simulink model "TenBots"  (R2016b)
settings: Solver=ode45  StartTime=0.0  StopTime=40  RelTol=1e-3  EnableMultiTasking=on
libraries: simulink x3
settings Model: Creator=Chris  LastModifiedBy=Syd
settings DataIOCC: LimitDataPoints=on  SaveFormat=Array
settings OptimizationCC: LifeSpan=inf
settings DebuggingCC: UnderspecifiedInitializationDetection=Classic  MergeDetectMultiDrivingBlocksExec=none  SolverPrmCheckMsg=warning  SFUnexpectedBacktrackingDiag=warning  SFNoUnconditionalDefaultTransitionDiag=warning  SFExecutionAtInitializationDiag=none
settings HardwareCC: ProdBitPerPointer=32  ProdBitPerSizeT=32  ProdBitPerPtrDiffT=32  ProdLargestAtomicFloat=None  ProdIntDivRoundTo=Undefined  ProdEndianess=Unspecified  ProdWordSize=32  ProdHWDeviceType=32-bit Generic
settings ModelReferenceCC: PropagateSignalLabelsOutOfModel=off
settings GRTTargetCC: TargetLangStandard=C89/C90 (ANSI)  GeneratePreprocessorConditionals=Disable all
settings ConfigComp: CovMetricSettings=dw  CovHtmlReporting=on  CovSaveCumulativeToWorkspaceVar=on  CovSaveSingleToWorkspaceVar=on  CovExternalEMLEnable=off

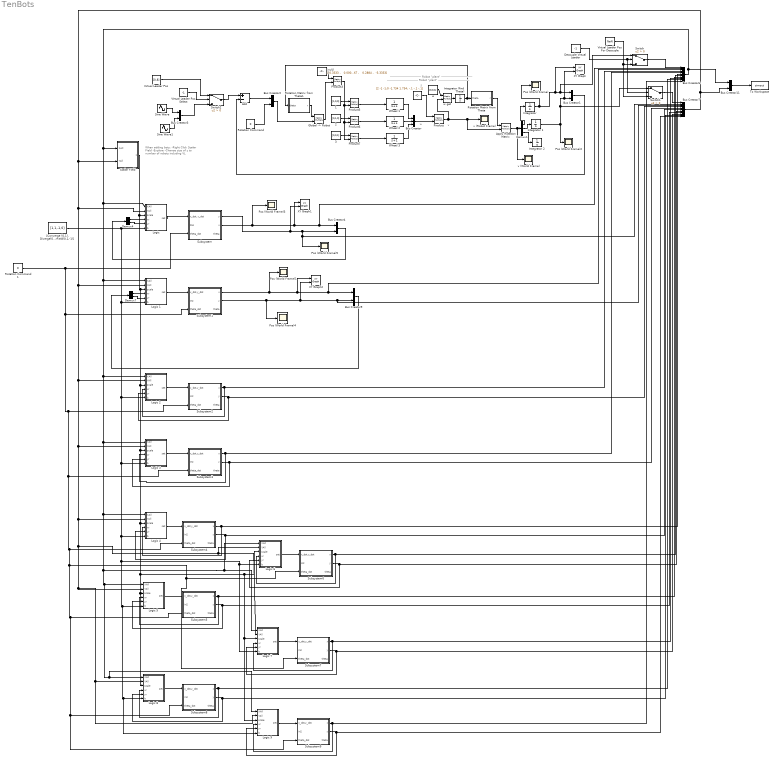
== system TenBots ==
  note: When adding bots:
      | -Right Click Scalar Field
      | -Explore
      | -Change size of z to number of robots including VL
  note: ------------------------------- Robot "plant" -------------------------------
  note: v
  note: w
  note: ------------------------------- Robot "plant" -------------------------------
  1 : Constant  Value=[1,0,0]  VectorParams1D=off
  2 : Constant  Value=[0,1,0]  VectorParams1D=off
  3 : Constant  Value=[0,0,1]  VectorParams1D=off
  Add : Sum  Inputs=+-
  Apply Rotation Matrix : Product  Multiplication=Matrix(*)
  Bus Creator : BusCreator  Inputs=3
  Bus Creator{1..4,9,11} (6 alike) : BusCreator  Inputs=2
  Bus Creator6 : BusCreator  Inputs=11
  Bus Creator7 : BusCreator  Inputs=11
  Decouple Virtual Leader : Constant  Value=-1
  Demux1 : Demux  Outputs=3
  Demux4 : Demux  Outputs=2
  Demux7 : Demux  Outputs=2
  "Global -> Robot" : Product  Multiplication=Matrix(*)
  "Integrator " : Integrator
  Integrator (find Theta) : Integrator
  Integrator 1 : Integrator
  Integrator 2 : Integrator  InitialCondition=1
  J : Constant  Value=[2 -1 -1;0 -1.734 1.734; -.1 -.1 -.1]
  "Logic " : MATLAB Function  TreatAsAtomicUnit=on
  Logic 1 : MATLAB Function  TreatAsAtomicUnit=on
  Logic 2 : MATLAB Function  TreatAsAtomicUnit=on
  Logic 3 : MATLAB Function  TreatAsAtomicUnit=on
  Logic 4 : MATLAB Function  TreatAsAtomicUnit=on
  Logic 5 : MATLAB Function  TreatAsAtomicUnit=on
  Logic 6 : MATLAB Function  TreatAsAtomicUnit=on
  Logic 7 : MATLAB Function  TreatAsAtomicUnit=on
  Logic 8 : MATLAB Function  TreatAsAtomicUnit=on
  Logic 9 : MATLAB Function  TreatAsAtomicUnit=on
  Pos (World Frame){,1..5} (6 alike) : Scope
  Product{,3,5..7} (5 alike) : Product  Multiplication=Matrix(*)
  Rotation Command : Constant  Value=0
  Rotation Command 1 : Constant  Value=0
  Rotation Matrix from Theta : MATLAB Function  TreatAsAtomicUnit=on
  Rotation Matrix from Theta1 : MATLAB Function  TreatAsAtomicUnit=on
  Scalar Field : MATLAB Function  TreatAsAtomicUnit=on
  Sine Wave : Sin  Amplitude=4  SampleTime=0
  Sine Wave1 : Sin  Phase=pi/2  SampleTime=0
  Subsystem : Subsystem
  Subsystem1 : Subsystem
  Subsystem2 : Subsystem
  Subsystem3 : Subsystem
  Subsystem4 : Subsystem
  Subsystem5 : Subsystem
  Subsystem6 : Subsystem
  Subsystem7 : Subsystem
  Subsystem8 : Subsystem
  Subsystem9 : Subsystem
  Switch : Switch  Criteria=u2 > Threshold
  Switch1 : Switch  Criteria=u2 > Threshold
  Switch2 : Switch  Criteria=u2 > Threshold
  To Workspace : ToWorkspace  VariableName=simout  SampleTime=-1
  VIrtual Leader Pos Select : Constant  Value=-1
  Virtual Leader Pos : Constant  Value=[0,8]
  Virtual Leader Pos For Decouple : Constant  Value=NaN
  Wheel 1 : TransferFcn  Denominator=[1 1]
  Wheel 2 : TransferFcn  Denominator=[1 1]
  Wheel 3 : TransferFcn  Denominator=[1 1]  ContinuousStateAttributes='orientation'
  XY Graph : simulink/Sinks/XY Graph  xmin=-1  xmax=3  ymin=-1  ymax=11  st=.1
  XY Graph1 : simulink/Sinks/XY Graph  xmin=-1  xmax=3  ymin=-1  ymax=10  st=.1
  XY Graph2 : simulink/Sinks/XY Graph  xmin=-1  xmax=3  ymin=-1  ymax=10  st=.1
  "[Converge (0,1), Diverge(0,1), Orbit(0,1,-1), ScalarField(0,1,-1)]" : Constant  Value=[1,1,-1,0]
  inv(J) : Constant  Value=|
      | [ 0.3333 ,   0.0000 ,  -3.3333
      |  ;  -0.1667  , -0.2884  , -3.3333
      |  ;  -0.1667 ,   0.2884 ,  -3.3333]
  v (Robot Frame) : Scope
  v (World Frame) : Scope
  w : Constant  Value=[0,0,1]  VectorParams1D=off
  w get : Product  Multiplication=Matrix(*)
  wires:
  Wheel 1/1 -> Bus Creator/1
  Wheel 3/1 -> Bus Creator/3
  J/1 -> Product/1
  Product/1 -> Apply Rotation Matrix/2, v (Robot Frame)/1, w get/2
  Product5/1 -> Wheel 1/1
  Product6/1 -> Wheel 2/1
  Product7/1 -> Wheel 3/1
  w get/1 -> Integrator (find Theta)/1
  Rotation Matrix from Theta/1(r) -> Apply Rotation Matrix/1
  Apply Rotation Matrix/1 -> Demux1/1, v (World Frame)/1
  inv(J)/1 -> Product3/1
  w/1 -> w get/1
  1/1 -> Product5/1
  Product3/1 -> Product6/2, Product7/2, Product5/2
  3/1 -> Product7/1
  2/1 -> Product6/1
  "Global -> Robot"/1 -> Product3/2
  Integrator (find Theta)/1 -> Rotation Matrix from Theta1/1(theta), Rotation Matrix from Theta/1(theta)
  Rotation Matrix from Theta1/1(r) -> "Global -> Robot"/1
  Bus Creator2/1 -> "Global -> Robot"/2
  Bus Creator/1 -> Product/2
  Wheel 2/1 -> Bus Creator/2
  Virtual Leader Pos/1 -> Switch2/1
  Integrator 1/1 -> Switch1/1, XY Graph/2, Bus Creator1/2, Pos (World Frame)2/1
  "Integrator "/1 -> XY Graph/1, Switch/1, Bus Creator1/1, Pos (World Frame)/1
  Bus Creator1/1 -> Add/2
  Add/1 -> Bus Creator2/1
  Demux1/1 -> "Integrator "/1
  Demux1/2 -> Integrator 1/1
  Demux1/3 -> Integrator 2/1
  Rotation Command/1 -> Bus Creator2/2
  Bus Creator4/1 -> Demux4/1
  Demux4/1 -> "Logic "/4(xr)
  Demux4/2 -> "Logic "/5(yr)
  Bus Creator9/1 -> Demux7/1
  Demux7/1 -> Logic 1/4(xr)
  Demux7/2 -> Logic 1/5(yr)
  Bus Creator11/1 -> To Workspace/1
  Subsystem/1(y) -> Bus Creator7/2, Pos (World Frame)5/1, Bus Creator4/2, XY Graph1/2
  Subsystem/2(x) -> Pos (World Frame)3/1, Bus Creator4/1, Bus Creator6/2, XY Graph1/1
  "Logic "/1(set) -> Subsystem/1("x_dot, y_dot")
  Subsystem1/1(x) -> Bus Creator9/1, Bus Creator6/3, XY Graph2/1, Pos (World Frame)1/1
  Subsystem1/2(y) -> Pos (World Frame)4/1, Bus Creator7/3, Bus Creator9/2, XY Graph2/2
  Logic 1/1(set) -> Subsystem1/1(x_dot,y_dot)
  Logic 2/1(set) -> Subsystem2/1(x_dot,y_dot)
  Subsystem2/1(x) -> Bus Creator6/4, Logic 2/4(xr)
  Subsystem2/2(y) -> Bus Creator7/4, Logic 2/5(yr)
  Logic 3/1(set) -> Subsystem3/1(x_dot,y_dot)
  Subsystem3/1(x) -> Logic 3/4(xr), Bus Creator6/5
  Subsystem3/2(y) -> Bus Creator7/5, Logic 3/5(yr)
  Switch/1 -> Bus Creator6/1
  Switch1/1 -> Bus Creator7/1
  Decouple Virtual Leader/1 -> Switch1/2, Switch/2
  Virtual Leader Pos For Decouple/1 -> Switch1/3, Switch/3
  Logic 4/1(set) -> Subsystem4/1(x_dot,y_dot)
  Subsystem4/1(x) -> Bus Creator6/6, Logic 4/4(xr)
  Subsystem4/2(y) -> Bus Creator7/6, Logic 4/5(yr)
  Logic 5/1(set) -> Subsystem5/1(x_dot,y_dot)
  Subsystem5/1(x) -> Bus Creator6/8, Logic 5/4(xr)
  Subsystem5/2(y) -> Bus Creator7/8, Logic 5/5(yr)
  Logic 6/1(set) -> Subsystem6/1(x_dot,y_dot)
  Subsystem6/1(x) -> Bus Creator6/7, Logic 6/4(xr)
  Subsystem6/2(y) -> Bus Creator7/7, Logic 6/5(yr)
  Logic 7/1(set) -> Subsystem7/1(x_dot,y_dot)
  Subsystem7/1(x) -> Bus Creator6/9, Logic 7/4(xr)
  Subsystem7/2(y) -> Bus Creator7/9, Logic 7/5(yr)
  Logic 8/1(set) -> Subsystem8/1(x_dot,y_dot)
  Subsystem8/1(x) -> Bus Creator6/10, Logic 8/4(xr)
  Subsystem8/2(y) -> Bus Creator7/10, Logic 8/5(yr)
  Bus Creator6/1 -> Bus Creator11/1, "Logic "/1(XAll), Logic 7/1(XAll), Logic 6/1(XAll), Logic 9/1(XAll), Logic 8/1(XAll), Logic 5/1(XAll), Logic 4/1(XAll), Logic 3/1(XAll), Logic 2/1(XAll), Logic 1/1(XAll), Scalar Field/1(XAll)
  Bus Creator7/1 -> Bus Creator11/2, "Logic "/2(YAll), Logic 7/2(YAll), Logic 6/2(YAll), Logic 9/2(YAll), Logic 8/2(YAll), Logic 5/2(YAll), Logic 4/2(YAll), Logic 3/2(YAll), Logic 2/2(YAll), Logic 1/2(YAll), Scalar Field/2(YAll)
  "[Converge (0,1), Diverge(0,1), Orbit(0,1,-1), ScalarField(0,1,-1)]"/1 -> "Logic "/6(b), Logic 2/6(b), Logic 7/6(b), Logic 6/6(b), Logic 9/6(b), Logic 8/6(b), Logic 5/6(b), Logic 4/6(b), Logic 3/6(b), Logic 1/6(b)
  Scalar Field/1(z) -> "Logic "/3(scale), Logic 9/3(scale), Logic 7/3(scale), Logic 6/3(scale), Logic 8/3(scale), Logic 5/3(scale), Logic 4/3(scale), Logic 3/3(scale), Logic 2/3(scale), Logic 1/3(scale)
  Logic 9/1(set) -> Subsystem9/1(x_dot,y_dot)
  Rotation Command 1/1 -> Subsystem7/3(theta_dot), Subsystem6/3(theta_dot), Subsystem9/3(theta_dot), Subsystem8/3(theta_dot), Subsystem5/3(theta_dot), Subsystem4/3(theta_dot), Subsystem3/3(theta_dot), Subsystem2/3(theta_dot), Subsystem1/3(theta_dot), Subsystem/3(theta_dot)
  Subsystem9/1(x) -> Bus Creator6/11, Logic 9/4(xr)
  Subsystem9/2(y) -> Bus Creator7/11, Logic 9/5(yr)
  Sine Wave/1 -> Bus Creator3/1
  Sine Wave1/1 -> Bus Creator3/2
  Switch2/1 -> Add/1
  Bus Creator3/1 -> Switch2/3
  VIrtual Leader Pos Select/1 -> Switch2/2

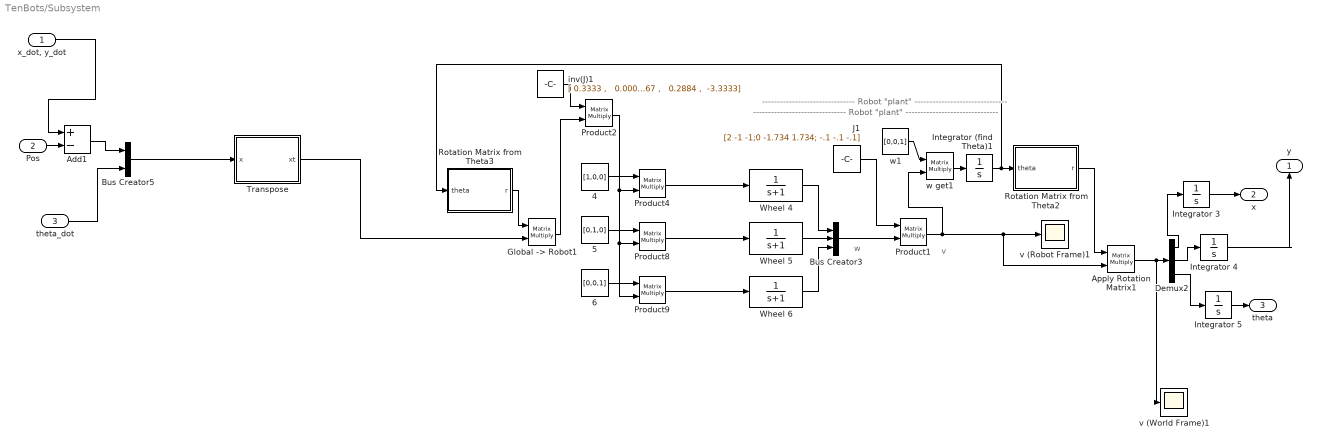
== system TenBots/Subsystem ==
  note: ------------------------------- Robot "plant" -------------------------------
  note: v
  note: w
  note: ------------------------------- Robot "plant" -------------------------------
  "x_dot, y_dot" : Inport
  Pos : Inport  Port=2
  theta_dot : Inport  Port=3
  4 : Constant  Value=[1,0,0]  VectorParams1D=off
  5 : Constant  Value=[0,1,0]  VectorParams1D=off
  6 : Constant  Value=[0,0,1]  VectorParams1D=off
  Add1 : Sum  Inputs=+-
  Apply Rotation Matrix1 : Product  Multiplication=Matrix(*)
  Bus Creator3 : BusCreator  Inputs=3
  Bus Creator5 : BusCreator  Inputs=2
  Demux2 : Demux  Outputs=3
  "Global -> Robot1" : Product  Multiplication=Matrix(*)
  Integrator (find Theta)1 : Integrator
  Integrator 3 : Integrator  InitialCondition=1
  Integrator 4 : Integrator  InitialCondition=1
  Integrator 5 : Integrator  InitialCondition=1
  J1 : Constant  Value=[2 -1 -1;0 -1.734 1.734; -.1 -.1 -.1]
  Product{1..2,4,8..9} (5 alike) : Product  Multiplication=Matrix(*)
  Rotation Matrix from Theta2 : MATLAB Function  TreatAsAtomicUnit=on
  Rotation Matrix from Theta3 : MATLAB Function  TreatAsAtomicUnit=on
  Transpose : MATLAB Function  TreatAsAtomicUnit=on
  Wheel 4 : TransferFcn  Denominator=[1 1]
  Wheel 5 : TransferFcn  Denominator=[1 1]
  Wheel 6 : TransferFcn  Denominator=[1 1]  ContinuousStateAttributes='orientation'
  inv(J)1 : Constant  Value=|
      | [ 0.3333 ,   0.0000 ,  -3.3333
      |  ;  -0.1667  , -0.2884  , -3.3333
      |  ;  -0.1667 ,   0.2884 ,  -3.3333]
  v (Robot Frame)1 : Scope
  v (World Frame)1 : Scope
  w get1 : Product  Multiplication=Matrix(*)
  w1 : Constant  Value=[0,0,1]  VectorParams1D=off
  y : Outport
  x : Outport  Port=2
  theta : Outport  Port=3
  wires:
  Product8/1 -> Wheel 5/1
  Product9/1 -> Wheel 6/1
  w get1/1 -> Integrator (find Theta)1/1
  Rotation Matrix from Theta2/1(r) -> Apply Rotation Matrix1/1
  Apply Rotation Matrix1/1 -> Demux2/1, v (World Frame)1/1
  Product1/1 -> Apply Rotation Matrix1/2, v (Robot Frame)1/1, w get1/2
  Product4/1 -> Wheel 4/1
  Wheel 6/1 -> Bus Creator3/3
  J1/1 -> Product1/1
  Wheel 4/1 -> Bus Creator3/1
  5/1 -> Product8/1
  Add1/1 -> Bus Creator5/1
  Demux2/2 -> Integrator 4/1
  Demux2/3 -> Integrator 5/1
  theta_dot/1 -> Bus Creator5/2
  Transpose/1(xt) -> "Global -> Robot1"/2
  4/1 -> Product4/1
  6/1 -> Product9/1
  Product2/1 -> Product8/2, Product9/2, Product4/2
  "x_dot, y_dot"/1 -> Add1/1
  Demux2/1 -> Integrator 3/1
  inv(J)1/1 -> Product2/1
  Integrator 3/1 -> x/1
  w1/1 -> w get1/1
  Bus Creator3/1 -> Product1/2
  Bus Creator5/1 -> Transpose/1(x)
  Integrator (find Theta)1/1 -> Rotation Matrix from Theta3/1(theta), Rotation Matrix from Theta2/1(theta)
  Wheel 5/1 -> Bus Creator3/2
  Integrator 4/1 -> y/1
  "Global -> Robot1"/1 -> Product2/2
  Rotation Matrix from Theta3/1(r) -> "Global -> Robot1"/1
  Pos/1 -> Add1/2
  Integrator 5/1 -> theta/1

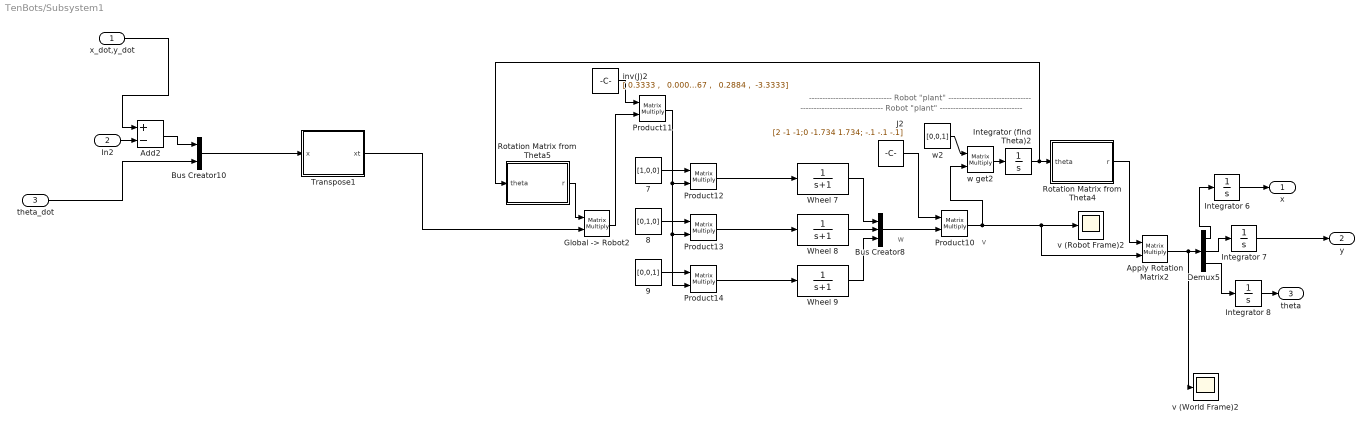
== system TenBots/Subsystem1 ==
  note: ------------------------------- Robot "plant" -------------------------------
  note: v
  note: w
  note: ------------------------------- Robot "plant" -------------------------------
  x_dot,y_dot : Inport
  In2 : Inport  Port=2
  theta_dot : Inport  Port=3
  7 : Constant  Value=[1,0,0]  VectorParams1D=off
  8 : Constant  Value=[0,1,0]  VectorParams1D=off
  9 : Constant  Value=[0,0,1]  VectorParams1D=off
  Add2 : Sum  Inputs=+-
  Apply Rotation Matrix2 : Product  Multiplication=Matrix(*)
  Bus Creator10 : BusCreator  Inputs=2
  Bus Creator8 : BusCreator  Inputs=3
  Demux5 : Demux  Outputs=3
  "Global -> Robot2" : Product  Multiplication=Matrix(*)
  Integrator (find Theta)2 : Integrator
  Integrator 6 : Integrator  InitialCondition=1
  Integrator 7 : Integrator  InitialCondition=2
  Integrator 8 : Integrator  InitialCondition=1
  J2 : Constant  Value=[2 -1 -1;0 -1.734 1.734; -.1 -.1 -.1]
  Product{10..14} (5 alike) : Product  Multiplication=Matrix(*)
  Rotation Matrix from Theta4 : MATLAB Function  TreatAsAtomicUnit=on
  Rotation Matrix from Theta5 : MATLAB Function  TreatAsAtomicUnit=on
  Transpose1 : MATLAB Function  TreatAsAtomicUnit=on
  Wheel 7 : TransferFcn  Denominator=[1 1]
  Wheel 8 : TransferFcn  Denominator=[1 1]
  Wheel 9 : TransferFcn  Denominator=[1 1]  ContinuousStateAttributes='orientation'
  inv(J)2 : Constant  Value=|
      | [ 0.3333 ,   0.0000 ,  -3.3333
      |  ;  -0.1667  , -0.2884  , -3.3333
      |  ;  -0.1667 ,   0.2884 ,  -3.3333]
  v (Robot Frame)2 : Scope
  v (World Frame)2 : Scope
  w get2 : Product  Multiplication=Matrix(*)
  w2 : Constant  Value=[0,0,1]  VectorParams1D=off
  x : Outport
  y : Outport  Port=2
  theta : Outport  Port=3
  wires:
  "Global -> Robot2"/1 -> Product11/2
  Bus Creator8/1 -> Product10/2
  Demux5/3 -> Integrator 8/1
  w get2/1 -> Integrator (find Theta)2/1
  theta_dot/1 -> Bus Creator10/2
  inv(J)2/1 -> Product11/1
  Integrator (find Theta)2/1 -> Rotation Matrix from Theta5/1(theta), Rotation Matrix from Theta4/1(theta)
  x_dot,y_dot/1 -> Add2/1
  Rotation Matrix from Theta5/1(r) -> "Global -> Robot2"/1
  J2/1 -> Product10/1
  Wheel 8/1 -> Bus Creator8/2
  Bus Creator10/1 -> Transpose1/1(x)
  Transpose1/1(xt) -> "Global -> Robot2"/2
  Product13/1 -> Wheel 8/1
  Product10/1 -> Apply Rotation Matrix2/2, v (Robot Frame)2/1, w get2/2
  Product14/1 -> Wheel 9/1
  w2/1 -> w get2/1
  Rotation Matrix from Theta4/1(r) -> Apply Rotation Matrix2/1
  Wheel 9/1 -> Bus Creator8/3
  Product12/1 -> Wheel 7/1
  Apply Rotation Matrix2/1 -> Demux5/1, v (World Frame)2/1
  Wheel 7/1 -> Bus Creator8/1
  7/1 -> Product12/1
  Integrator 7/1 -> y/1
  Add2/1 -> Bus Creator10/1
  Demux5/1 -> Integrator 6/1
  Integrator 6/1 -> x/1
  Product11/1 -> Product13/2, Product14/2, Product12/2
  9/1 -> Product14/1
  8/1 -> Product13/1
  Demux5/2 -> Integrator 7/1
  In2/1 -> Add2/2
  Integrator 8/1 -> theta/1

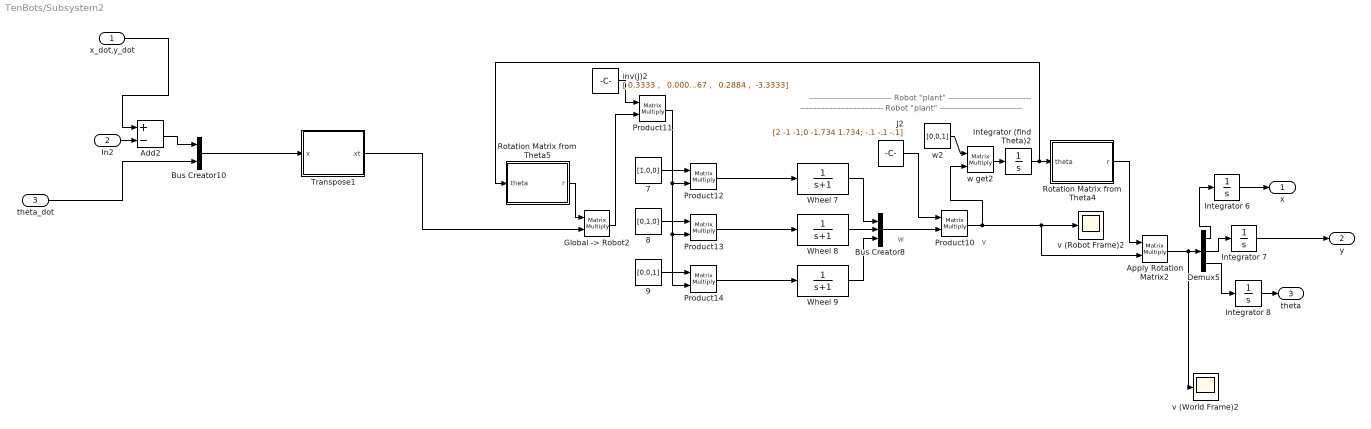
== system TenBots/Subsystem2 ==
  note: ------------------------------- Robot "plant" -------------------------------
  note: v
  note: w
  note: ------------------------------- Robot "plant" -------------------------------
  x_dot,y_dot : Inport
  In2 : Inport  Port=2
  theta_dot : Inport  Port=3
  7 : Constant  Value=[1,0,0]  VectorParams1D=off
  8 : Constant  Value=[0,1,0]  VectorParams1D=off
  9 : Constant  Value=[0,0,1]  VectorParams1D=off
  Add2 : Sum  Inputs=+-
  Apply Rotation Matrix2 : Product  Multiplication=Matrix(*)
  Bus Creator10 : BusCreator  Inputs=2
  Bus Creator8 : BusCreator  Inputs=3
  Demux5 : Demux  Outputs=3
  "Global -> Robot2" : Product  Multiplication=Matrix(*)
  Integrator (find Theta)2 : Integrator
  Integrator 6 : Integrator  InitialCondition=2
  Integrator 7 : Integrator  InitialCondition=1
  Integrator 8 : Integrator  InitialCondition=1
  J2 : Constant  Value=[2 -1 -1;0 -1.734 1.734; -.1 -.1 -.1]
  Product{10..14} (5 alike) : Product  Multiplication=Matrix(*)
  Rotation Matrix from Theta4 : MATLAB Function  TreatAsAtomicUnit=on
  Rotation Matrix from Theta5 : MATLAB Function  TreatAsAtomicUnit=on
  Transpose1 : MATLAB Function  TreatAsAtomicUnit=on
  Wheel 7 : TransferFcn  Denominator=[1 1]
  Wheel 8 : TransferFcn  Denominator=[1 1]
  Wheel 9 : TransferFcn  Denominator=[1 1]  ContinuousStateAttributes='orientation'
  inv(J)2 : Constant  Value=|
      | [ 0.3333 ,   0.0000 ,  -3.3333
      |  ;  -0.1667  , -0.2884  , -3.3333
      |  ;  -0.1667 ,   0.2884 ,  -3.3333]
  v (Robot Frame)2 : Scope
  v (World Frame)2 : Scope
  w get2 : Product  Multiplication=Matrix(*)
  w2 : Constant  Value=[0,0,1]  VectorParams1D=off
  x : Outport
  y : Outport  Port=2
  theta : Outport  Port=3
  wires:
  "Global -> Robot2"/1 -> Product11/2
  Bus Creator8/1 -> Product10/2
  Demux5/3 -> Integrator 8/1
  w get2/1 -> Integrator (find Theta)2/1
  theta_dot/1 -> Bus Creator10/2
  inv(J)2/1 -> Product11/1
  Integrator (find Theta)2/1 -> Rotation Matrix from Theta5/1(theta), Rotation Matrix from Theta4/1(theta)
  x_dot,y_dot/1 -> Add2/1
  Rotation Matrix from Theta5/1(r) -> "Global -> Robot2"/1
  J2/1 -> Product10/1
  Wheel 8/1 -> Bus Creator8/2
  Bus Creator10/1 -> Transpose1/1(x)
  Transpose1/1(xt) -> "Global -> Robot2"/2
  Product13/1 -> Wheel 8/1
  Product10/1 -> Apply Rotation Matrix2/2, v (Robot Frame)2/1, w get2/2
  Product14/1 -> Wheel 9/1
  w2/1 -> w get2/1
  Rotation Matrix from Theta4/1(r) -> Apply Rotation Matrix2/1
  Wheel 9/1 -> Bus Creator8/3
  Product12/1 -> Wheel 7/1
  Apply Rotation Matrix2/1 -> Demux5/1, v (World Frame)2/1
  Wheel 7/1 -> Bus Creator8/1
  7/1 -> Product12/1
  Integrator 7/1 -> y/1
  Add2/1 -> Bus Creator10/1
  Demux5/1 -> Integrator 6/1
  Integrator 6/1 -> x/1
  Product11/1 -> Product13/2, Product14/2, Product12/2
  9/1 -> Product14/1
  8/1 -> Product13/1
  Demux5/2 -> Integrator 7/1
  In2/1 -> Add2/2
  Integrator 8/1 -> theta/1

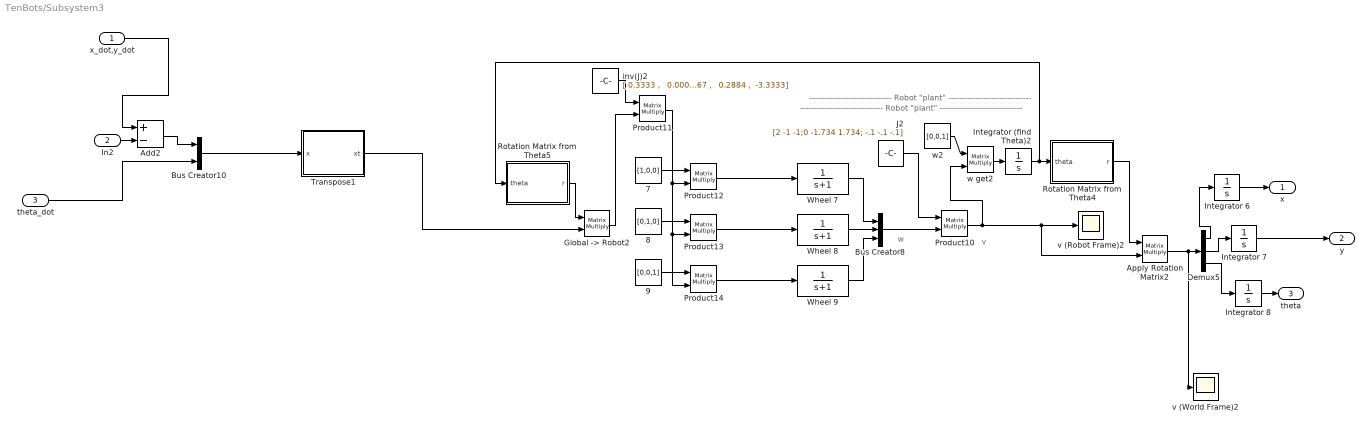
== system TenBots/Subsystem3 ==
  note: ------------------------------- Robot "plant" -------------------------------
  note: v
  note: w
  note: ------------------------------- Robot "plant" -------------------------------
  x_dot,y_dot : Inport
  In2 : Inport  Port=2
  theta_dot : Inport  Port=3
  7 : Constant  Value=[1,0,0]  VectorParams1D=off
  8 : Constant  Value=[0,1,0]  VectorParams1D=off
  9 : Constant  Value=[0,0,1]  VectorParams1D=off
  Add2 : Sum  Inputs=+-
  Apply Rotation Matrix2 : Product  Multiplication=Matrix(*)
  Bus Creator10 : BusCreator  Inputs=2
  Bus Creator8 : BusCreator  Inputs=3
  Demux5 : Demux  Outputs=3
  "Global -> Robot2" : Product  Multiplication=Matrix(*)
  Integrator (find Theta)2 : Integrator
  Integrator 6 : Integrator  InitialCondition=2
  Integrator 7 : Integrator  InitialCondition=2
  Integrator 8 : Integrator  InitialCondition=1
  J2 : Constant  Value=[2 -1 -1;0 -1.734 1.734; -.1 -.1 -.1]
  Product{10..14} (5 alike) : Product  Multiplication=Matrix(*)
  Rotation Matrix from Theta4 : MATLAB Function  TreatAsAtomicUnit=on
  Rotation Matrix from Theta5 : MATLAB Function  TreatAsAtomicUnit=on
  Transpose1 : MATLAB Function  TreatAsAtomicUnit=on
  Wheel 7 : TransferFcn  Denominator=[1 1]
  Wheel 8 : TransferFcn  Denominator=[1 1]
  Wheel 9 : TransferFcn  Denominator=[1 1]  ContinuousStateAttributes='orientation'
  inv(J)2 : Constant  Value=|
      | [ 0.3333 ,   0.0000 ,  -3.3333
      |  ;  -0.1667  , -0.2884  , -3.3333
      |  ;  -0.1667 ,   0.2884 ,  -3.3333]
  v (Robot Frame)2 : Scope
  v (World Frame)2 : Scope
  w get2 : Product  Multiplication=Matrix(*)
  w2 : Constant  Value=[0,0,1]  VectorParams1D=off
  x : Outport
  y : Outport  Port=2
  theta : Outport  Port=3
  wires:
  "Global -> Robot2"/1 -> Product11/2
  Bus Creator8/1 -> Product10/2
  Demux5/3 -> Integrator 8/1
  w get2/1 -> Integrator (find Theta)2/1
  theta_dot/1 -> Bus Creator10/2
  inv(J)2/1 -> Product11/1
  Integrator (find Theta)2/1 -> Rotation Matrix from Theta5/1(theta), Rotation Matrix from Theta4/1(theta)
  x_dot,y_dot/1 -> Add2/1
  Rotation Matrix from Theta5/1(r) -> "Global -> Robot2"/1
  J2/1 -> Product10/1
  Wheel 8/1 -> Bus Creator8/2
  Bus Creator10/1 -> Transpose1/1(x)
  Transpose1/1(xt) -> "Global -> Robot2"/2
  Product13/1 -> Wheel 8/1
  Product10/1 -> Apply Rotation Matrix2/2, v (Robot Frame)2/1, w get2/2
  Product14/1 -> Wheel 9/1
  w2/1 -> w get2/1
  Rotation Matrix from Theta4/1(r) -> Apply Rotation Matrix2/1
  Wheel 9/1 -> Bus Creator8/3
  Product12/1 -> Wheel 7/1
  Apply Rotation Matrix2/1 -> Demux5/1, v (World Frame)2/1
  Wheel 7/1 -> Bus Creator8/1
  7/1 -> Product12/1
  Integrator 7/1 -> y/1
  Add2/1 -> Bus Creator10/1
  Demux5/1 -> Integrator 6/1
  Integrator 6/1 -> x/1
  Product11/1 -> Product13/2, Product14/2, Product12/2
  9/1 -> Product14/1
  8/1 -> Product13/1
  Demux5/2 -> Integrator 7/1
  In2/1 -> Add2/2
  Integrator 8/1 -> theta/1

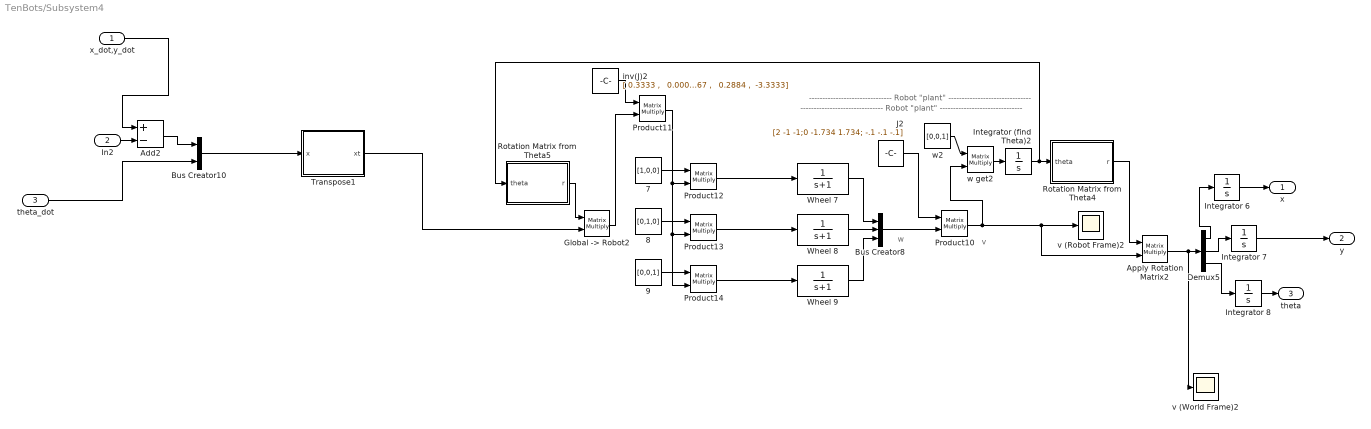
== system TenBots/Subsystem4 ==
  note: ------------------------------- Robot "plant" -------------------------------
  note: v
  note: w
  note: ------------------------------- Robot "plant" -------------------------------
  x_dot,y_dot : Inport
  In2 : Inport  Port=2
  theta_dot : Inport  Port=3
  7 : Constant  Value=[1,0,0]  VectorParams1D=off
  8 : Constant  Value=[0,1,0]  VectorParams1D=off
  9 : Constant  Value=[0,0,1]  VectorParams1D=off
  Add2 : Sum  Inputs=+-
  Apply Rotation Matrix2 : Product  Multiplication=Matrix(*)
  Bus Creator10 : BusCreator  Inputs=2
  Bus Creator8 : BusCreator  Inputs=3
  Demux5 : Demux  Outputs=3
  "Global -> Robot2" : Product  Multiplication=Matrix(*)
  Integrator (find Theta)2 : Integrator
  Integrator 6 : Integrator  InitialCondition=3
  Integrator 7 : Integrator
  Integrator 8 : Integrator  InitialCondition=1
  J2 : Constant  Value=[2 -1 -1;0 -1.734 1.734; -.1 -.1 -.1]
  Product{10..14} (5 alike) : Product  Multiplication=Matrix(*)
  Rotation Matrix from Theta4 : MATLAB Function  TreatAsAtomicUnit=on
  Rotation Matrix from Theta5 : MATLAB Function  TreatAsAtomicUnit=on
  Transpose1 : MATLAB Function  TreatAsAtomicUnit=on
  Wheel 7 : TransferFcn  Denominator=[1 1]
  Wheel 8 : TransferFcn  Denominator=[1 1]
  Wheel 9 : TransferFcn  Denominator=[1 1]  ContinuousStateAttributes='orientation'
  inv(J)2 : Constant  Value=|
      | [ 0.3333 ,   0.0000 ,  -3.3333
      |  ;  -0.1667  , -0.2884  , -3.3333
      |  ;  -0.1667 ,   0.2884 ,  -3.3333]
  v (Robot Frame)2 : Scope
  v (World Frame)2 : Scope
  w get2 : Product  Multiplication=Matrix(*)
  w2 : Constant  Value=[0,0,1]  VectorParams1D=off
  x : Outport
  y : Outport  Port=2
  theta : Outport  Port=3
  wires:
  "Global -> Robot2"/1 -> Product11/2
  Bus Creator8/1 -> Product10/2
  Demux5/3 -> Integrator 8/1
  w get2/1 -> Integrator (find Theta)2/1
  theta_dot/1 -> Bus Creator10/2
  inv(J)2/1 -> Product11/1
  Integrator (find Theta)2/1 -> Rotation Matrix from Theta5/1(theta), Rotation Matrix from Theta4/1(theta)
  x_dot,y_dot/1 -> Add2/1
  Rotation Matrix from Theta5/1(r) -> "Global -> Robot2"/1
  J2/1 -> Product10/1
  Wheel 8/1 -> Bus Creator8/2
  Bus Creator10/1 -> Transpose1/1(x)
  Transpose1/1(xt) -> "Global -> Robot2"/2
  Product13/1 -> Wheel 8/1
  Product10/1 -> Apply Rotation Matrix2/2, v (Robot Frame)2/1, w get2/2
  Product14/1 -> Wheel 9/1
  w2/1 -> w get2/1
  Rotation Matrix from Theta4/1(r) -> Apply Rotation Matrix2/1
  Wheel 9/1 -> Bus Creator8/3
  Product12/1 -> Wheel 7/1
  Apply Rotation Matrix2/1 -> Demux5/1, v (World Frame)2/1
  Wheel 7/1 -> Bus Creator8/1
  7/1 -> Product12/1
  Integrator 7/1 -> y/1
  Add2/1 -> Bus Creator10/1
  Demux5/1 -> Integrator 6/1
  Integrator 6/1 -> x/1
  Product11/1 -> Product13/2, Product14/2, Product12/2
  9/1 -> Product14/1
  8/1 -> Product13/1
  Demux5/2 -> Integrator 7/1
  In2/1 -> Add2/2
  Integrator 8/1 -> theta/1

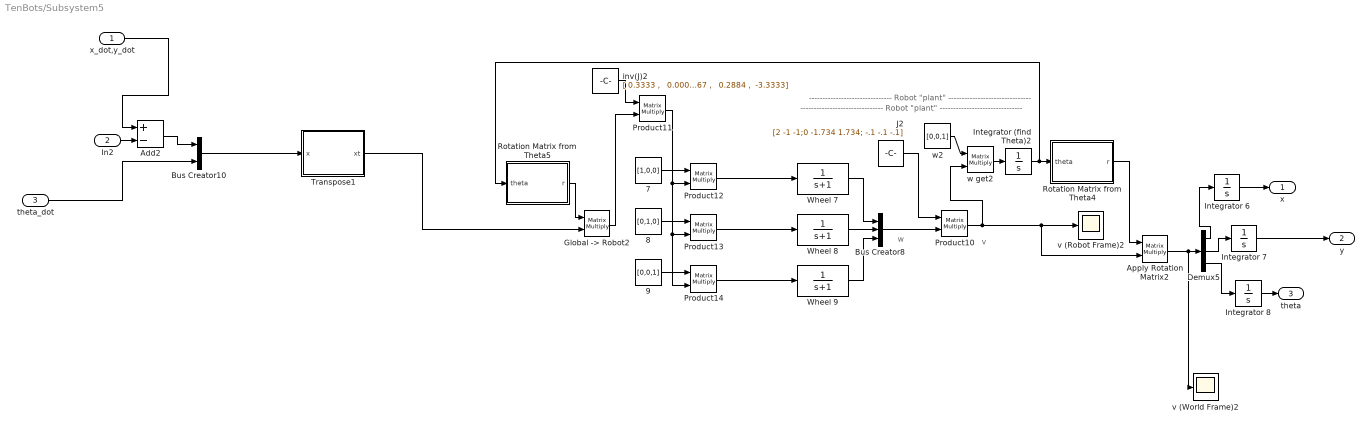
== system TenBots/Subsystem5 ==
  note: ------------------------------- Robot "plant" -------------------------------
  note: v
  note: w
  note: ------------------------------- Robot "plant" -------------------------------
  x_dot,y_dot : Inport
  In2 : Inport  Port=2
  theta_dot : Inport  Port=3
  7 : Constant  Value=[1,0,0]  VectorParams1D=off
  8 : Constant  Value=[0,1,0]  VectorParams1D=off
  9 : Constant  Value=[0,0,1]  VectorParams1D=off
  Add2 : Sum  Inputs=+-
  Apply Rotation Matrix2 : Product  Multiplication=Matrix(*)
  Bus Creator10 : BusCreator  Inputs=2
  Bus Creator8 : BusCreator  Inputs=3
  Demux5 : Demux  Outputs=3
  "Global -> Robot2" : Product  Multiplication=Matrix(*)
  Integrator (find Theta)2 : Integrator
  Integrator 6 : Integrator  InitialCondition=1
  Integrator 7 : Integrator
  Integrator 8 : Integrator  InitialCondition=1
  J2 : Constant  Value=[2 -1 -1;0 -1.734 1.734; -.1 -.1 -.1]
  Product{10..14} (5 alike) : Product  Multiplication=Matrix(*)
  Rotation Matrix from Theta4 : MATLAB Function  TreatAsAtomicUnit=on
  Rotation Matrix from Theta5 : MATLAB Function  TreatAsAtomicUnit=on
  Transpose1 : MATLAB Function  TreatAsAtomicUnit=on
  Wheel 7 : TransferFcn  Denominator=[1 1]
  Wheel 8 : TransferFcn  Denominator=[1 1]
  Wheel 9 : TransferFcn  Denominator=[1 1]  ContinuousStateAttributes='orientation'
  inv(J)2 : Constant  Value=|
      | [ 0.3333 ,   0.0000 ,  -3.3333
      |  ;  -0.1667  , -0.2884  , -3.3333
      |  ;  -0.1667 ,   0.2884 ,  -3.3333]
  v (Robot Frame)2 : Scope
  v (World Frame)2 : Scope
  w get2 : Product  Multiplication=Matrix(*)
  w2 : Constant  Value=[0,0,1]  VectorParams1D=off
  x : Outport
  y : Outport  Port=2
  theta : Outport  Port=3
  wires:
  "Global -> Robot2"/1 -> Product11/2
  Bus Creator8/1 -> Product10/2
  Demux5/3 -> Integrator 8/1
  w get2/1 -> Integrator (find Theta)2/1
  theta_dot/1 -> Bus Creator10/2
  inv(J)2/1 -> Product11/1
  Integrator (find Theta)2/1 -> Rotation Matrix from Theta5/1(theta), Rotation Matrix from Theta4/1(theta)
  x_dot,y_dot/1 -> Add2/1
  Rotation Matrix from Theta5/1(r) -> "Global -> Robot2"/1
  J2/1 -> Product10/1
  Wheel 8/1 -> Bus Creator8/2
  Bus Creator10/1 -> Transpose1/1(x)
  Transpose1/1(xt) -> "Global -> Robot2"/2
  Product13/1 -> Wheel 8/1
  Product10/1 -> Apply Rotation Matrix2/2, v (Robot Frame)2/1, w get2/2
  Product14/1 -> Wheel 9/1
  w2/1 -> w get2/1
  Rotation Matrix from Theta4/1(r) -> Apply Rotation Matrix2/1
  Wheel 9/1 -> Bus Creator8/3
  Product12/1 -> Wheel 7/1
  Apply Rotation Matrix2/1 -> Demux5/1, v (World Frame)2/1
  Wheel 7/1 -> Bus Creator8/1
  7/1 -> Product12/1
  Integrator 7/1 -> y/1
  Add2/1 -> Bus Creator10/1
  Demux5/1 -> Integrator 6/1
  Integrator 6/1 -> x/1
  Product11/1 -> Product13/2, Product14/2, Product12/2
  9/1 -> Product14/1
  8/1 -> Product13/1
  Demux5/2 -> Integrator 7/1
  In2/1 -> Add2/2
  Integrator 8/1 -> theta/1

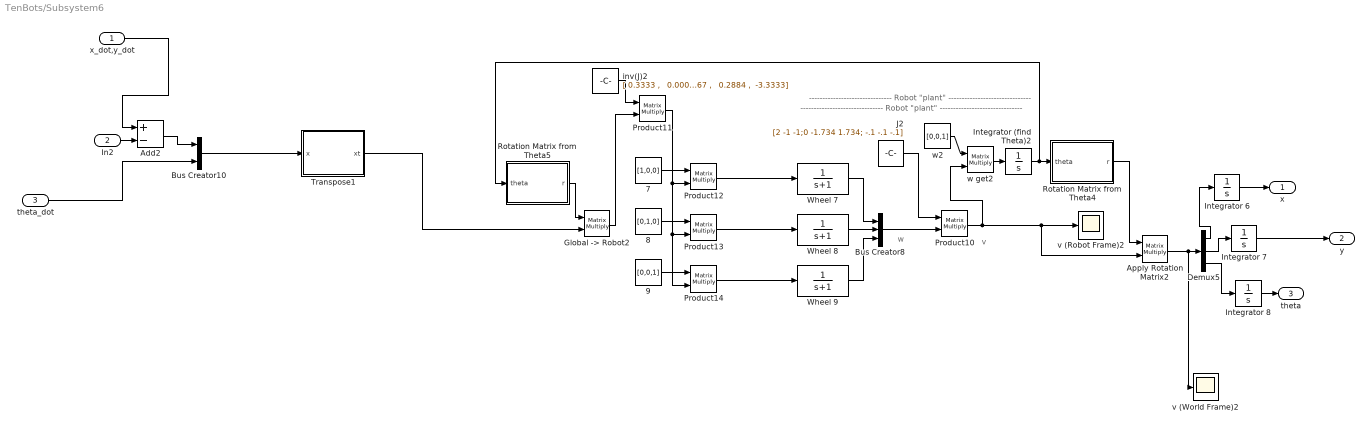
== system TenBots/Subsystem6 ==
  note: ------------------------------- Robot "plant" -------------------------------
  note: v
  note: w
  note: ------------------------------- Robot "plant" -------------------------------
  x_dot,y_dot : Inport
  In2 : Inport  Port=2
  theta_dot : Inport  Port=3
  7 : Constant  Value=[1,0,0]  VectorParams1D=off
  8 : Constant  Value=[0,1,0]  VectorParams1D=off
  9 : Constant  Value=[0,0,1]  VectorParams1D=off
  Add2 : Sum  Inputs=+-
  Apply Rotation Matrix2 : Product  Multiplication=Matrix(*)
  Bus Creator10 : BusCreator  Inputs=2
  Bus Creator8 : BusCreator  Inputs=3
  Demux5 : Demux  Outputs=3
  "Global -> Robot2" : Product  Multiplication=Matrix(*)
  Integrator (find Theta)2 : Integrator
  Integrator 6 : Integrator  InitialCondition=2
  Integrator 7 : Integrator
  Integrator 8 : Integrator  InitialCondition=1
  J2 : Constant  Value=[2 -1 -1;0 -1.734 1.734; -.1 -.1 -.1]
  Product{10..14} (5 alike) : Product  Multiplication=Matrix(*)
  Rotation Matrix from Theta4 : MATLAB Function  TreatAsAtomicUnit=on
  Rotation Matrix from Theta5 : MATLAB Function  TreatAsAtomicUnit=on
  Transpose1 : MATLAB Function  TreatAsAtomicUnit=on
  Wheel 7 : TransferFcn  Denominator=[1 1]
  Wheel 8 : TransferFcn  Denominator=[1 1]
  Wheel 9 : TransferFcn  Denominator=[1 1]  ContinuousStateAttributes='orientation'
  inv(J)2 : Constant  Value=|
      | [ 0.3333 ,   0.0000 ,  -3.3333
      |  ;  -0.1667  , -0.2884  , -3.3333
      |  ;  -0.1667 ,   0.2884 ,  -3.3333]
  v (Robot Frame)2 : Scope
  v (World Frame)2 : Scope
  w get2 : Product  Multiplication=Matrix(*)
  w2 : Constant  Value=[0,0,1]  VectorParams1D=off
  x : Outport
  y : Outport  Port=2
  theta : Outport  Port=3
  wires:
  "Global -> Robot2"/1 -> Product11/2
  Bus Creator8/1 -> Product10/2
  Demux5/3 -> Integrator 8/1
  w get2/1 -> Integrator (find Theta)2/1
  theta_dot/1 -> Bus Creator10/2
  inv(J)2/1 -> Product11/1
  Integrator (find Theta)2/1 -> Rotation Matrix from Theta5/1(theta), Rotation Matrix from Theta4/1(theta)
  x_dot,y_dot/1 -> Add2/1
  Rotation Matrix from Theta5/1(r) -> "Global -> Robot2"/1
  J2/1 -> Product10/1
  Wheel 8/1 -> Bus Creator8/2
  Bus Creator10/1 -> Transpose1/1(x)
  Transpose1/1(xt) -> "Global -> Robot2"/2
  Product13/1 -> Wheel 8/1
  Product10/1 -> Apply Rotation Matrix2/2, v (Robot Frame)2/1, w get2/2
  Product14/1 -> Wheel 9/1
  w2/1 -> w get2/1
  Rotation Matrix from Theta4/1(r) -> Apply Rotation Matrix2/1
  Wheel 9/1 -> Bus Creator8/3
  Product12/1 -> Wheel 7/1
  Apply Rotation Matrix2/1 -> Demux5/1, v (World Frame)2/1
  Wheel 7/1 -> Bus Creator8/1
  7/1 -> Product12/1
  Integrator 7/1 -> y/1
  Add2/1 -> Bus Creator10/1
  Demux5/1 -> Integrator 6/1
  Integrator 6/1 -> x/1
  Product11/1 -> Product13/2, Product14/2, Product12/2
  9/1 -> Product14/1
  8/1 -> Product13/1
  Demux5/2 -> Integrator 7/1
  In2/1 -> Add2/2
  Integrator 8/1 -> theta/1

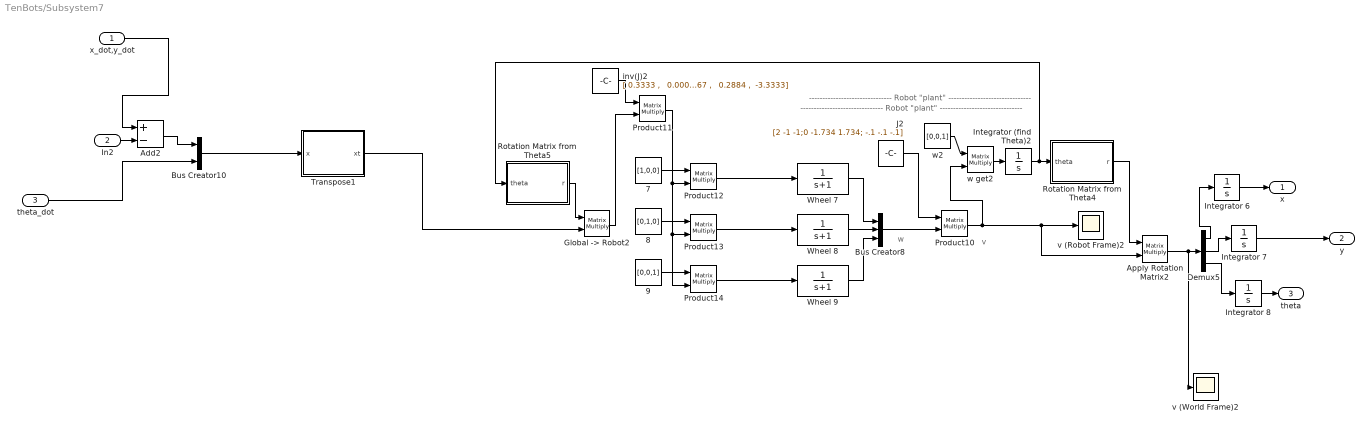
== system TenBots/Subsystem7 ==
  note: ------------------------------- Robot "plant" -------------------------------
  note: v
  note: w
  note: ------------------------------- Robot "plant" -------------------------------
  x_dot,y_dot : Inport
  In2 : Inport  Port=2
  theta_dot : Inport  Port=3
  7 : Constant  Value=[1,0,0]  VectorParams1D=off
  8 : Constant  Value=[0,1,0]  VectorParams1D=off
  9 : Constant  Value=[0,0,1]  VectorParams1D=off
  Add2 : Sum  Inputs=+-
  Apply Rotation Matrix2 : Product  Multiplication=Matrix(*)
  Bus Creator10 : BusCreator  Inputs=2
  Bus Creator8 : BusCreator  Inputs=3
  Demux5 : Demux  Outputs=3
  "Global -> Robot2" : Product  Multiplication=Matrix(*)
  Integrator (find Theta)2 : Integrator
  Integrator 6 : Integrator  InitialCondition=1
  Integrator 7 : Integrator  InitialCondition=-1
  Integrator 8 : Integrator  InitialCondition=1
  J2 : Constant  Value=[2 -1 -1;0 -1.734 1.734; -.1 -.1 -.1]
  Product{10..14} (5 alike) : Product  Multiplication=Matrix(*)
  Rotation Matrix from Theta4 : MATLAB Function  TreatAsAtomicUnit=on
  Rotation Matrix from Theta5 : MATLAB Function  TreatAsAtomicUnit=on
  Transpose1 : MATLAB Function  TreatAsAtomicUnit=on
  Wheel 7 : TransferFcn  Denominator=[1 1]
  Wheel 8 : TransferFcn  Denominator=[1 1]
  Wheel 9 : TransferFcn  Denominator=[1 1]  ContinuousStateAttributes='orientation'
  inv(J)2 : Constant  Value=|
      | [ 0.3333 ,   0.0000 ,  -3.3333
      |  ;  -0.1667  , -0.2884  , -3.3333
      |  ;  -0.1667 ,   0.2884 ,  -3.3333]
  v (Robot Frame)2 : Scope
  v (World Frame)2 : Scope
  w get2 : Product  Multiplication=Matrix(*)
  w2 : Constant  Value=[0,0,1]  VectorParams1D=off
  x : Outport
  y : Outport  Port=2
  theta : Outport  Port=3
  wires:
  "Global -> Robot2"/1 -> Product11/2
  Bus Creator8/1 -> Product10/2
  Demux5/3 -> Integrator 8/1
  w get2/1 -> Integrator (find Theta)2/1
  theta_dot/1 -> Bus Creator10/2
  inv(J)2/1 -> Product11/1
  Integrator (find Theta)2/1 -> Rotation Matrix from Theta5/1(theta), Rotation Matrix from Theta4/1(theta)
  x_dot,y_dot/1 -> Add2/1
  Rotation Matrix from Theta5/1(r) -> "Global -> Robot2"/1
  J2/1 -> Product10/1
  Wheel 8/1 -> Bus Creator8/2
  Bus Creator10/1 -> Transpose1/1(x)
  Transpose1/1(xt) -> "Global -> Robot2"/2
  Product13/1 -> Wheel 8/1
  Product10/1 -> Apply Rotation Matrix2/2, v (Robot Frame)2/1, w get2/2
  Product14/1 -> Wheel 9/1
  w2/1 -> w get2/1
  Rotation Matrix from Theta4/1(r) -> Apply Rotation Matrix2/1
  Wheel 9/1 -> Bus Creator8/3
  Product12/1 -> Wheel 7/1
  Apply Rotation Matrix2/1 -> Demux5/1, v (World Frame)2/1
  Wheel 7/1 -> Bus Creator8/1
  7/1 -> Product12/1
  Integrator 7/1 -> y/1
  Add2/1 -> Bus Creator10/1
  Demux5/1 -> Integrator 6/1
  Integrator 6/1 -> x/1
  Product11/1 -> Product13/2, Product14/2, Product12/2
  9/1 -> Product14/1
  8/1 -> Product13/1
  Demux5/2 -> Integrator 7/1
  In2/1 -> Add2/2
  Integrator 8/1 -> theta/1

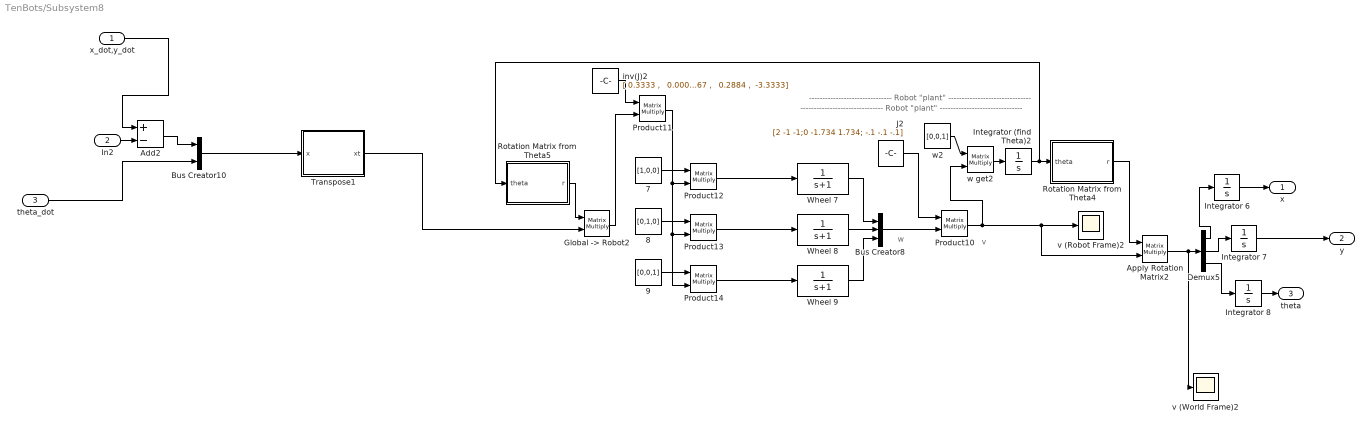
== system TenBots/Subsystem8 ==
  note: ------------------------------- Robot "plant" -------------------------------
  note: v
  note: w
  note: ------------------------------- Robot "plant" -------------------------------
  x_dot,y_dot : Inport
  In2 : Inport  Port=2
  theta_dot : Inport  Port=3
  7 : Constant  Value=[1,0,0]  VectorParams1D=off
  8 : Constant  Value=[0,1,0]  VectorParams1D=off
  9 : Constant  Value=[0,0,1]  VectorParams1D=off
  Add2 : Sum  Inputs=+-
  Apply Rotation Matrix2 : Product  Multiplication=Matrix(*)
  Bus Creator10 : BusCreator  Inputs=2
  Bus Creator8 : BusCreator  Inputs=3
  Demux5 : Demux  Outputs=3
  "Global -> Robot2" : Product  Multiplication=Matrix(*)
  Integrator (find Theta)2 : Integrator
  Integrator 6 : Integrator  InitialCondition=2
  Integrator 7 : Integrator  InitialCondition=-1
  Integrator 8 : Integrator  InitialCondition=1
  J2 : Constant  Value=[2 -1 -1;0 -1.734 1.734; -.1 -.1 -.1]
  Product{10..14} (5 alike) : Product  Multiplication=Matrix(*)
  Rotation Matrix from Theta4 : MATLAB Function  TreatAsAtomicUnit=on
  Rotation Matrix from Theta5 : MATLAB Function  TreatAsAtomicUnit=on
  Transpose1 : MATLAB Function  TreatAsAtomicUnit=on
  Wheel 7 : TransferFcn  Denominator=[1 1]
  Wheel 8 : TransferFcn  Denominator=[1 1]
  Wheel 9 : TransferFcn  Denominator=[1 1]  ContinuousStateAttributes='orientation'
  inv(J)2 : Constant  Value=|
      | [ 0.3333 ,   0.0000 ,  -3.3333
      |  ;  -0.1667  , -0.2884  , -3.3333
      |  ;  -0.1667 ,   0.2884 ,  -3.3333]
  v (Robot Frame)2 : Scope
  v (World Frame)2 : Scope
  w get2 : Product  Multiplication=Matrix(*)
  w2 : Constant  Value=[0,0,1]  VectorParams1D=off
  x : Outport
  y : Outport  Port=2
  theta : Outport  Port=3
  wires:
  "Global -> Robot2"/1 -> Product11/2
  Bus Creator8/1 -> Product10/2
  Demux5/3 -> Integrator 8/1
  w get2/1 -> Integrator (find Theta)2/1
  theta_dot/1 -> Bus Creator10/2
  inv(J)2/1 -> Product11/1
  Integrator (find Theta)2/1 -> Rotation Matrix from Theta5/1(theta), Rotation Matrix from Theta4/1(theta)
  x_dot,y_dot/1 -> Add2/1
  Rotation Matrix from Theta5/1(r) -> "Global -> Robot2"/1
  J2/1 -> Product10/1
  Wheel 8/1 -> Bus Creator8/2
  Bus Creator10/1 -> Transpose1/1(x)
  Transpose1/1(xt) -> "Global -> Robot2"/2
  Product13/1 -> Wheel 8/1
  Product10/1 -> Apply Rotation Matrix2/2, v (Robot Frame)2/1, w get2/2
  Product14/1 -> Wheel 9/1
  w2/1 -> w get2/1
  Rotation Matrix from Theta4/1(r) -> Apply Rotation Matrix2/1
  Wheel 9/1 -> Bus Creator8/3
  Product12/1 -> Wheel 7/1
  Apply Rotation Matrix2/1 -> Demux5/1, v (World Frame)2/1
  Wheel 7/1 -> Bus Creator8/1
  7/1 -> Product12/1
  Integrator 7/1 -> y/1
  Add2/1 -> Bus Creator10/1
  Demux5/1 -> Integrator 6/1
  Integrator 6/1 -> x/1
  Product11/1 -> Product13/2, Product14/2, Product12/2
  9/1 -> Product14/1
  8/1 -> Product13/1
  Demux5/2 -> Integrator 7/1
  In2/1 -> Add2/2
  Integrator 8/1 -> theta/1

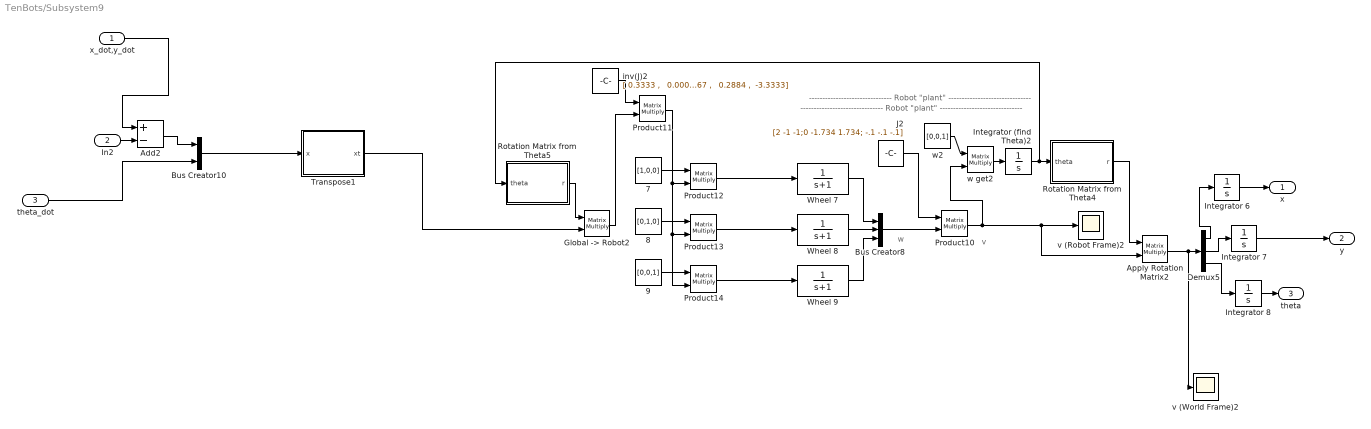
== system TenBots/Subsystem9 ==
  note: ------------------------------- Robot "plant" -------------------------------
  note: v
  note: w
  note: ------------------------------- Robot "plant" -------------------------------
  x_dot,y_dot : Inport
  In2 : Inport  Port=2
  theta_dot : Inport  Port=3
  7 : Constant  Value=[1,0,0]  VectorParams1D=off
  8 : Constant  Value=[0,1,0]  VectorParams1D=off
  9 : Constant  Value=[0,0,1]  VectorParams1D=off
  Add2 : Sum  Inputs=+-
  Apply Rotation Matrix2 : Product  Multiplication=Matrix(*)
  Bus Creator10 : BusCreator  Inputs=2
  Bus Creator8 : BusCreator  Inputs=3
  Demux5 : Demux  Outputs=3
  "Global -> Robot2" : Product  Multiplication=Matrix(*)
  Integrator (find Theta)2 : Integrator
  Integrator 6 : Integrator  InitialCondition=3
  Integrator 7 : Integrator  InitialCondition=-1
  Integrator 8 : Integrator  InitialCondition=1
  J2 : Constant  Value=[2 -1 -1;0 -1.734 1.734; -.1 -.1 -.1]
  Product{10..14} (5 alike) : Product  Multiplication=Matrix(*)
  Rotation Matrix from Theta4 : MATLAB Function  TreatAsAtomicUnit=on
  Rotation Matrix from Theta5 : MATLAB Function  TreatAsAtomicUnit=on
  Transpose1 : MATLAB Function  TreatAsAtomicUnit=on
  Wheel 7 : TransferFcn  Denominator=[1 1]
  Wheel 8 : TransferFcn  Denominator=[1 1]
  Wheel 9 : TransferFcn  Denominator=[1 1]  ContinuousStateAttributes='orientation'
  inv(J)2 : Constant  Value=|
      | [ 0.3333 ,   0.0000 ,  -3.3333
      |  ;  -0.1667  , -0.2884  , -3.3333
      |  ;  -0.1667 ,   0.2884 ,  -3.3333]
  v (Robot Frame)2 : Scope
  v (World Frame)2 : Scope
  w get2 : Product  Multiplication=Matrix(*)
  w2 : Constant  Value=[0,0,1]  VectorParams1D=off
  x : Outport
  y : Outport  Port=2
  theta : Outport  Port=3
  wires:
  "Global -> Robot2"/1 -> Product11/2
  Bus Creator8/1 -> Product10/2
  Demux5/3 -> Integrator 8/1
  w get2/1 -> Integrator (find Theta)2/1
  theta_dot/1 -> Bus Creator10/2
  inv(J)2/1 -> Product11/1
  Integrator (find Theta)2/1 -> Rotation Matrix from Theta5/1(theta), Rotation Matrix from Theta4/1(theta)
  x_dot,y_dot/1 -> Add2/1
  Rotation Matrix from Theta5/1(r) -> "Global -> Robot2"/1
  J2/1 -> Product10/1
  Wheel 8/1 -> Bus Creator8/2
  Bus Creator10/1 -> Transpose1/1(x)
  Transpose1/1(xt) -> "Global -> Robot2"/2
  Product13/1 -> Wheel 8/1
  Product10/1 -> Apply Rotation Matrix2/2, v (Robot Frame)2/1, w get2/2
  Product14/1 -> Wheel 9/1
  w2/1 -> w get2/1
  Rotation Matrix from Theta4/1(r) -> Apply Rotation Matrix2/1
  Wheel 9/1 -> Bus Creator8/3
  Product12/1 -> Wheel 7/1
  Apply Rotation Matrix2/1 -> Demux5/1, v (World Frame)2/1
  Wheel 7/1 -> Bus Creator8/1
  7/1 -> Product12/1
  Integrator 7/1 -> y/1
  Add2/1 -> Bus Creator10/1
  Demux5/1 -> Integrator 6/1
  Integrator 6/1 -> x/1
  Product11/1 -> Product13/2, Product14/2, Product12/2
  9/1 -> Product14/1
  8/1 -> Product13/1
  Demux5/2 -> Integrator 7/1
  In2/1 -> Add2/2
  Integrator 8/1 -> theta/1

== matlab function TenBots/Rotation Matrix from Theta1 ==
  data: theta input; r output
function r = fcn(theta)

r =[cos(theta) sin(theta),0; -sin(theta) cos(theta),0;0,0,1];

== matlab function TenBots/Rotation Matrix from Theta ==
  data: theta input; r output
function r = fcn(theta)

r =[cos(theta) -sin(theta),0; sin(theta) cos(theta),0;0,0,1];

== matlab function TenBots/Subsystem/Rotation Matrix from Theta2 ==
  data: theta input; r output
function r = fcn(theta)

r =[cos(theta) -sin(theta),0; sin(theta) cos(theta),0;0,0,1];

== matlab function TenBots/Subsystem/Rotation Matrix from Theta3 ==
  data: theta input; r output
function r = fcn(theta)

r =[cos(theta) sin(theta),0; -sin(theta) cos(theta),0;0,0,1];

== matlab function TenBots/Logic  ==
  data: XAll input; set output; YAll input; scale input; xr input; yr input; b input
function set = f(XAll,YAll,scale,xr,yr,b)
set = swarmlogic(XAll,YAll,scale,xr,yr,b);

== matlab function TenBots/Subsystem/Transpose ==
  data: x input; xt output
function xt = fcn(x)

xt=x.';

== matlab function TenBots/Logic 1 ==
  data: XAll input; set output; YAll input; scale input; xr input; yr input; b input
function set = f(XAll,YAll,scale,xr,yr,b)
set = swarmlogic(XAll,YAll,scale,xr,yr,b);

== matlab function TenBots/Subsystem1/Rotation Matrix from Theta4 ==
  data: theta input; r output
function r = fcn(theta)

r =[cos(theta) -sin(theta),0; sin(theta) cos(theta),0;0,0,1];

== matlab function TenBots/Subsystem1/Rotation Matrix from Theta5 ==
  data: theta input; r output
function r = fcn(theta)

r =[cos(theta) sin(theta),0; -sin(theta) cos(theta),0;0,0,1];

== matlab function TenBots/Subsystem1/Transpose1 ==
  data: x input; xt output
function xt = fcn(x)

xt=x.';

== matlab function TenBots/Scalar Field ==
  data: XAll input; z output size=[1 11]; YAll input
function z = fcn(XAll,YAll)
%coder.varsize('z',[1,length(XAll)]);
z=zeros(1,length(XAll));
for i = 1:length(XAll)
    z(i)=sqrt(XAll(i)^2+YAll(i)^2);  %<--define scalar field
end

== matlab function TenBots/Logic 2 ==
  data: XAll input; set output; YAll input; scale input; xr input; yr input; b input
function set = f(XAll,YAll,scale,xr,yr,b)
set = swarmlogic(XAll,YAll,scale,xr,yr,b);

== matlab function TenBots/Subsystem2/Rotation Matrix from Theta4 ==
  data: theta input; r output
function r = fcn(theta)

r =[cos(theta) -sin(theta),0; sin(theta) cos(theta),0;0,0,1];

== matlab function TenBots/Subsystem2/Rotation Matrix from Theta5 ==
  data: theta input; r output
function r = fcn(theta)

r =[cos(theta) sin(theta),0; -sin(theta) cos(theta),0;0,0,1];

== matlab function TenBots/Subsystem2/Transpose1 ==
  data: x input; xt output
function xt = fcn(x)

xt=x.';

== matlab function TenBots/Logic 3 ==
  data: XAll input; set output; YAll input; scale input; xr input; yr input; b input
function set = f(XAll,YAll,scale,xr,yr,b)
set = swarmlogic(XAll,YAll,scale,xr,yr,b);

== matlab function TenBots/Subsystem3/Rotation Matrix from Theta4 ==
  data: theta input; r output
function r = fcn(theta)

r =[cos(theta) -sin(theta),0; sin(theta) cos(theta),0;0,0,1];

== matlab function TenBots/Subsystem3/Rotation Matrix from Theta5 ==
  data: theta input; r output
function r = fcn(theta)

r =[cos(theta) sin(theta),0; -sin(theta) cos(theta),0;0,0,1];

== matlab function TenBots/Subsystem3/Transpose1 ==
  data: x input; xt output
function xt = fcn(x)

xt=x.';

== matlab function TenBots/Logic 4 ==
  data: XAll input; set output; YAll input; scale input; xr input; yr input; b input
function set = f(XAll,YAll,scale,xr,yr,b)
set = swarmlogic(XAll,YAll,scale,xr,yr,b);

== matlab function TenBots/Subsystem4/Rotation Matrix from Theta4 ==
  data: theta input; r output
function r = fcn(theta)

r =[cos(theta) -sin(theta),0; sin(theta) cos(theta),0;0,0,1];

== matlab function TenBots/Subsystem4/Rotation Matrix from Theta5 ==
  data: theta input; r output
function r = fcn(theta)

r =[cos(theta) sin(theta),0; -sin(theta) cos(theta),0;0,0,1];

== matlab function TenBots/Subsystem4/Transpose1 ==
  data: x input; xt output
function xt = fcn(x)

xt=x.';

== matlab function TenBots/Logic 5 ==
  data: XAll input; set output; YAll input; scale input; xr input; yr input; b input
function set = f(XAll,YAll,scale,xr,yr,b)
set = swarmlogic(XAll,YAll,scale,xr,yr,b);

== matlab function TenBots/Subsystem5/Rotation Matrix from Theta4 ==
  data: theta input; r output
function r = fcn(theta)

r =[cos(theta) -sin(theta),0; sin(theta) cos(theta),0;0,0,1];

== matlab function TenBots/Subsystem5/Rotation Matrix from Theta5 ==
  data: theta input; r output
function r = fcn(theta)

r =[cos(theta) sin(theta),0; -sin(theta) cos(theta),0;0,0,1];

== matlab function TenBots/Subsystem5/Transpose1 ==
  data: x input; xt output
function xt = fcn(x)

xt=x.';

== matlab function TenBots/Logic 6 ==
  data: XAll input; set output; YAll input; scale input; xr input; yr input; b input
function set = f(XAll,YAll,scale,xr,yr,b)
set = swarmlogic(XAll,YAll,scale,xr,yr,b);

== matlab function TenBots/Subsystem6/Rotation Matrix from Theta4 ==
  data: theta input; r output
function r = fcn(theta)

r =[cos(theta) -sin(theta),0; sin(theta) cos(theta),0;0,0,1];

== matlab function TenBots/Subsystem6/Rotation Matrix from Theta5 ==
  data: theta input; r output
function r = fcn(theta)

r =[cos(theta) sin(theta),0; -sin(theta) cos(theta),0;0,0,1];

== matlab function TenBots/Subsystem6/Transpose1 ==
  data: x input; xt output
function xt = fcn(x)

xt=x.';

== matlab function TenBots/Logic 7 ==
  data: XAll input; set output; YAll input; scale input; xr input; yr input; b input
function set = f(XAll,YAll,scale,xr,yr,b)
set = swarmlogic(XAll,YAll,scale,xr,yr,b);

== matlab function TenBots/Subsystem7/Rotation Matrix from Theta4 ==
  data: theta input; r output
function r = fcn(theta)

r =[cos(theta) -sin(theta),0; sin(theta) cos(theta),0;0,0,1];

== matlab function TenBots/Subsystem7/Rotation Matrix from Theta5 ==
  data: theta input; r output
function r = fcn(theta)

r =[cos(theta) sin(theta),0; -sin(theta) cos(theta),0;0,0,1];

== matlab function TenBots/Subsystem7/Transpose1 ==
  data: x input; xt output
function xt = fcn(x)

xt=x.';

== matlab function TenBots/Logic 8 ==
  data: XAll input; set output; YAll input; scale input; xr input; yr input; b input
function set = f(XAll,YAll,scale,xr,yr,b)
set = swarmlogic(XAll,YAll,scale,xr,yr,b);

== matlab function TenBots/Subsystem8/Rotation Matrix from Theta4 ==
  data: theta input; r output
function r = fcn(theta)

r =[cos(theta) -sin(theta),0; sin(theta) cos(theta),0;0,0,1];

== matlab function TenBots/Subsystem8/Rotation Matrix from Theta5 ==
  data: theta input; r output
function r = fcn(theta)

r =[cos(theta) sin(theta),0; -sin(theta) cos(theta),0;0,0,1];

== matlab function TenBots/Subsystem8/Transpose1 ==
  data: x input; xt output
function xt = fcn(x)

xt=x.';

== matlab function TenBots/Logic 9 ==
  data: XAll input; set output; YAll input; scale input; xr input; yr input; b input
function set = f(XAll,YAll,scale,xr,yr,b)
set = swarmlogic(XAll,YAll,scale,xr,yr,b);

== matlab function TenBots/Subsystem9/Rotation Matrix from Theta4 ==
  data: theta input; r output
function r = fcn(theta)

r =[cos(theta) -sin(theta),0; sin(theta) cos(theta),0;0,0,1];

== matlab function TenBots/Subsystem9/Rotation Matrix from Theta5 ==
  data: theta input; r output
function r = fcn(theta)

r =[cos(theta) sin(theta),0; -sin(theta) cos(theta),0;0,0,1];

== matlab function TenBots/Subsystem9/Transpose1 ==
  data: x input; xt output
function xt = fcn(x)

xt=x.';
